simulink model "final_LIithium_inductionmotor_powered_vehicle"  (R2020a)
settings: Solver=VariableStepAuto  StartTime=0  StopTime=240  RelTol=1e-3
libraries: autolibshared x4, autolibdatasheetbattery x1, autolibim x1, simulink x1, autolibmotorctrlr x1, autolibinverter x1, autolibshareddiff x1, autolibsharedcoupling x1
(part 1 of 3)
settings Model: Creator=User  LastModifiedBy=User

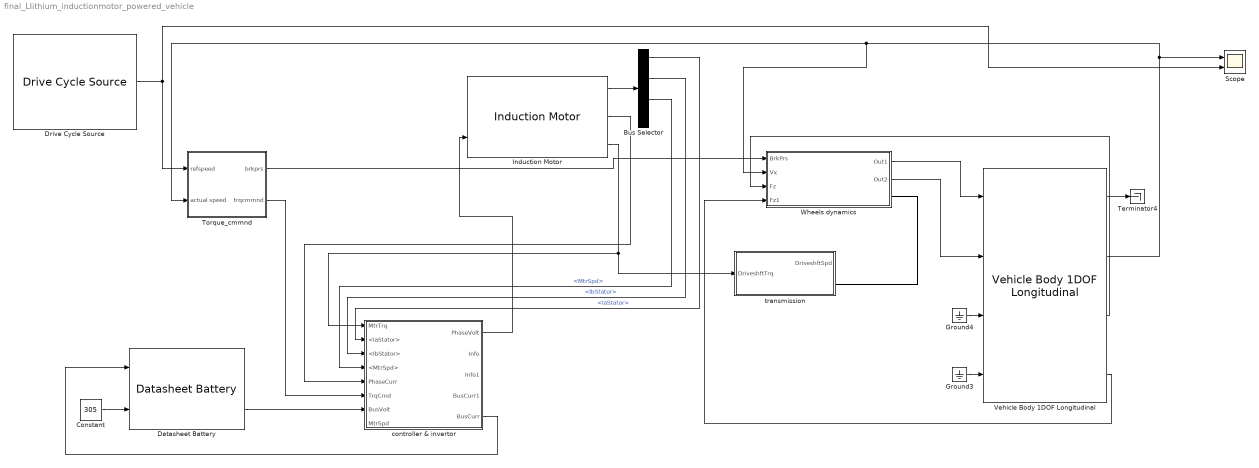
== system final_LIithium_inductionmotor_powered_vehicle ==
  Bus Selector : BusSelector  OutputSignals=IaStator,IbStator,MtrSpd,PwrInfo.PwrTrnsfrd.PwrMtr
  Constant : Constant  Value=305
  Datasheet Battery : autolibdatasheetbattery/Datasheet Battery  CapacityCtrl=Parameter  OutputVlt=Filtered  BattChargeMax=100  Em=[2.8 3.228 3.284 3.361 3.408 3.427 3.472 3.477 3.493 3.504 3.516 3.528 3.537 3.545 3.555 3.561 3.566 3.576 3.587 3.589 3.594 3.6 3.608 3.61 3.616 3.619 3.626 3.632 3.637 3.64 3.645 3.646 3.652 3.655 3.658 3.661 3.664 3.668 3.673 3.678 3.68 3.681 3.686 3.692 3.699 3.702 3.705 3.71 3.717 3.723 3.728 3.733 3.735 3.742 3.749 3.755 3.761 3.768 3.773 3.78 3.791 3.798 3.798 3.814 3.818 3.825 3.841 3.846 3.855 3.863 3.877 3.885 3.894 3.907 3.919 3.926 3.935 3.944 3.954 3.964 3.974 3.988 3.998 4.014 4.029 4.034 4.047 4.065 4.074 4.086 4.097 4.131 4.126 4.138 4.15 4.18 4.174 4.187 4.207 4.231 4.221]  CapLUTBp=[0 0.01 0.02 0.03 0.04 0.05 0.06 0.07 0.08 0.09 0.1 0.11 0.12 0.13 0.14 0.15 0.16 0.17 0.18 0.19 0.2 0.21 0.22 0.23 0.24 0.25 0.26 0.27 0.28 0.29 0.3 0.31 0.32 0.33 0.34 0.35 0.36 0.37 0.38 0.39 0.4 0.41 0.42 0.43 0.44 0.45 0.46 0.47 0.48 0.49 0.5 0.51 0.52 0.53 0.54 0.55 0.56 0.57 0.58 0.59 0.6 0.61 0.62 0.63 0.64 0.65 0.66 0.67 0.68 0.69 0.7 0.71 0.72 0.73 0.74 0.75 0.76 0.77 0.78 0.79 0.8 0.81 0.82 0.83 0.84 0.85 0.86 0.87 0.88 0.89 0.9 0.91 0.92 0.93 0.94 0.95 0.96 0.97 0.98 0.99 1]  RInt=[0.008846 0.009319 0.009027 0.00847 0.01032 0.01314;0.006389 0.006554 0.005553 0.005525 0.006043 0.007805;0.004364 0.004101 0.00406 0.003452 0.003846 0.004517;0.002031 0.002563 0.002532 0.00246 0.002716 0.003047;0.001443 0.001825 0.001795 0.001778 0.001924 0.002234;0.0005603 0.0007192 0.0006887 0.0007557 0.0007355 0.001014;0.001028 0.001338 0.001 0.001536 0.001546 0.002789]  BattTempBp=[243.1 253.1 263.1 273.1 283.1 298.1 313.1]  CapSOCBp=[0 0.2 0.4 0.6 0.8 1]  Ns=1  Np=1  BattCapInit=100  Tc=1/1000  Vinit=500  RefBlkName='autolibdatasheetbattery/Datasheet Battery'
      settings: SourceProductName=Powertrain Blockset
  Drive Cycle Source : autolibshared/Drive Cycle Source  cycleVar=IM240  fileVar=cycleFTP75.mat  tfinal="240  seconds"  cycleRepeat=off  outAccPort=off  outGearPort=off  gearList=No gear data  t_wot1=5  xdot_woto=0  xdot_wot1=30  t_wot2=20  xdot_wot2=0  t_wotend=30  srcUnit=m/s  outUnit=m/s  srcAccUnit=m/s/s  outAccUnit=m/s^2  dt=0  aMode=1  faultOption=off  velBnd=2  velBndUnit=mph  inUnit=m/s  timeBnd=1  failOption=off  stopSim=off  maxFaultCnt=10  maxFaultTime=2  maxTotFaultTime=15  traceOption=off  dtTrace=1  traceWindow=10  lastDCname=IM240 Inspection & Maintenance Driving Schedule Velocity  lastOutUnit=mph  lastDT=0  lastTB=1  lastSB=2  forceCalcBound=off
      settings: SourceProductBaseCode=PW,MT,VE,VP
  Ground3 : Ground
  Ground4 : Ground
  Induction Motor : autolibim/Induction Motor  sim_type=Continuous  Ts=0.001  port_config=Speed  Zs=[1.77 0.0139]  Zr="[1.34  0.0121]"  Lm=0.3687  P=4  theta_init=0  omega_init=0  mechanical=[0.001 0 0]  RefBlkName='autolibim/Induction Motor'
      settings: SourceProductBaseCode=PW,MT,VE,VP
  Scope : Scope  NumInputPorts=2
  Terminator4 : Terminator
  Torque_cmmnd : Subsystem
  Vehicle Body 1DOF Longitudinal : autolibshared/Vehicle Body 1DOF Longitudinal  VariantControl=SL  extFMode=off  extMMode=off  extTamb=off  wind3D=off  aMode=aMode  NF=2  NR=2  m=2200  a=1.4  b=1.8  h=.35  Cd=.3  Cl=0  Cpm=0  Af=4  x_o=0  xdot_o=0  Pabs=101325  T=273  g=9.81
      settings: SourceProductBaseCode=PW
  Wheels dynamics : Subsystem
  controller & invertor : Subsystem
  transmission : Subsystem
  wires:
  Induction Motor/1 -> Bus Selector/1
  Constant/1 -> Datasheet Battery/2
  Induction Motor/3 -> controller & invertor/1(MtrTrq), transmission/1(DriveshftTrq)
  Vehicle Body 1DOF Longitudinal/2 -> Scope/1, Wheels dynamics/2(Vx), Torque_cmmnd/2(actual speed)
  Vehicle Body 1DOF Longitudinal/1 -> Terminator4/1
  Ground4/1 -> Vehicle Body 1DOF Longitudinal/3
  Ground3/1 -> Vehicle Body 1DOF Longitudinal/4
  Drive Cycle Source/1 -> Torque_cmmnd/1(refspeed), Scope/2
  Vehicle Body 1DOF Longitudinal/3 -> Wheels dynamics/3(Fz)
  Vehicle Body 1DOF Longitudinal/4 -> Wheels dynamics/4(Fz1)
  Wheels dynamics/1(Out1) -> Vehicle Body 1DOF Longitudinal/1
  Wheels dynamics/2(Out2) -> Vehicle Body 1DOF Longitudinal/2
  Bus Selector/1 -> controller & invertor/2(<IaStator>)  "<IaStator>"
  Bus Selector/2 -> controller & invertor/3(<IbStator>)  "<IbStator>"
  Bus Selector/3 -> controller & invertor/4(<MtrSpd>)  "<MtrSpd>"
  Induction Motor/2 -> controller & invertor/5(PhaseCurr)
  Datasheet Battery/2 -> controller & invertor/7(BusVolt)
  controller & invertor/1(PhaseVolt) -> Induction Motor/2
  controller & invertor/5(BusCurr) -> Datasheet Battery/1
  Torque_cmmnd/1(brkprs) -> Wheels dynamics/1(BrkPrs)
  Torque_cmmnd/2(trqcmmnd) -> controller & invertor/6(TrqCmd)
  connections:
  Wheels dynamics/RConn1 -- transmission/RConn1

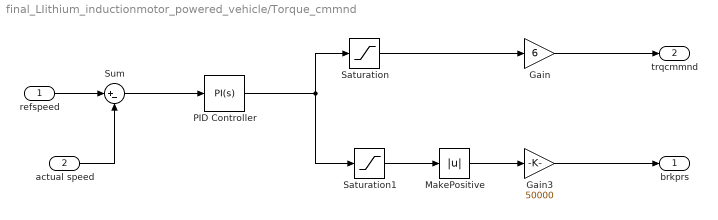
== system final_LIithium_inductionmotor_powered_vehicle/Torque_cmmnd ==
  refspeed : Inport
  actual speed : Inport  Port=2
  Gain : Gain  Gain=6
  Gain3 : Gain  Gain=50000
  MakePositive : Abs
  PID Controller : simulink/Continuous/PID Controller  Controller=PI  Form=Parallel  TimeDomain=Continuous-time  UseExternalTs=off  SampleTime=-1  IntegratorMethod=Forward Euler  FilterMethod=Forward Euler  ControllerParametersSource=internal  P=30  I=0.09  D=0  UseFilter=on  N=100  TunerSelectOption=Transfer Function Based (PID Tuner App)  InitialConditionSource=internal  InitialConditionForIntegrator=0  InitialConditionForFilter=0  DifferentiatorICPrevScaledInput=0  ExternalReset=none  TrackingMode=off  Kt=1  LimitOutput=on  UpperSaturationLimit=600  LowerSaturationLimit=-2000  LinearizeAsGain=on  AntiWindupMode=none  Kb=1  POutMin=[]  POutMax=[]  IOutMin=[]  IOutMax=[]  DOutMin=[]  DOutMax=[]  NOutMin=[]  NOutMax=[]  SumOutMin=[]  SumOutMax=[]  SaturationOutMin=[]  SaturationOutMax=[]  PParamMin=[]  PParamMax=[]  IParamMin=[]  IParamMax=[]  DParamMin=[]  DParamMax=[]  NParamMin=[]  NParamMax=[]  KbParamMin=[]  KbParamMax=[]  KtParamMin=[]  KtParamMax=[]  KbOutMin=[]  KbOutMax=[]  KtOutMin=[]  KtOutMax=[]  IntegratorOutMin=[]  IntegratorOutMax=[]  FilterOutMin=[]  FilterOutMax=[]  SumI1OutMin=[]  SumI1OutMax=[]  SumI2OutMin=[]  SumI2OutMax=[]  SumI3OutMin=[]  SumI3OutMax=[]  SumI4OutMin=[]  SumI4OutMax=[]  SumDOutMin=[]  SumDOutMax=[]  DifferentiatorOutMin=[]  DifferentiatorOutMax=[]  FilterDiffOutCoefMin=[]  FilterDiffOutCoefMax=[]  ReciprocalOutMin=[]  ReciprocalOutMax=[]  SumDenOutMin=[]  SumDenOutMax=[]  SumNumOutMin=[]  SumNumOutMax=[]  DivideOutMin=[]  DivideOutMax=[]  UdiffTsProdOutMin=[]  UdiffTsProdOutMax=[]  NTsProdOutMin=[]  NTsProdOutMax=[]  UintegralTsProdOutMin=[]  UintegralTsProdOutMax=[]  UngainTsProdOutMin=[]  UngainTsProdOutMax=[]  IntegratorContinuousStateAttributes=''  IntegratorStateMustResolveToSignalObject=off  IntegratorRTWStateStorageClass=Auto  FilterContinuousStateAttributes=''  FilterStateMustResolveToSignalObject=off  FilterRTWStateStorageClass=Auto  ParallelPVariant=InternalParameters  IdealPVariant=Disabled  IVariant=InternalParameters  DVariant=Disabled  IntegratorVariant=Continuous  SatVariant=Enabled  AWVariant=Passthrough  PCopyVariant=Disabled  TRVariant=Disabled  FdbkBlocksVariant=Forward  IdealPFdbkVariant=Disabled  SatFdbkVariant=Disabled  DerivativeFilterVariant=Disabled  NVariant=Disabled  NCopyVariant=Disabled_SignalSpec  FilterICVariant=Disabled  IntegratorICVariant=InternalICs  ExternalResetVariant=Disabled  TRSumVariant=Passthrough  SumFdbkVariant=Disabled  SumVariant=Sum_PI  TsampFilterVariant=InternalTs  TsampNgainVariant=Passthrough  TsampIntegralVariant=Passthrough
  Saturation : Saturate  UpperLimit=100  LowerLimit=0
  Saturation1 : Saturate  UpperLimit=0  LowerLimit=-100
  Sum : Sum  Inputs=|+-
  brkprs : Outport
  trqcmmnd : Outport  Port=2
  wires:
  refspeed/1 -> Sum/1
  MakePositive/1 -> Gain3/1
  PID Controller/1 -> Saturation1/1, Saturation/1
  Gain3/1 -> brkprs/1
  Sum/1 -> PID Controller/1
  Saturation1/1 -> MakePositive/1
  actual speed/1 -> Sum/2
  Saturation/1 -> Gain/1
  Gain/1 -> trqcmmnd/1
